simulink model "MotionControlRobuFastObsDynWithPredAdams2"  (Simulink 7.1)
settings: Solver=ode23  StartTime=0.0  StopTime=50  MaxStep=0.002  MinStep=0.0001  RelTol=0.2  AbsTol=0.1
StartFcn:
  | parameters
StopFcn:
  | replay
values from neighbouring files (symbols this model uses):
  ADAMS_cwd = '/home/roland/Bureau/Simulateur/SimulateurAdamsFaizRobuFASTB2'    [Controls_Plant_1.m]
  ADAMS_exec = ''    [Controls_Plant_1.m]
  ADAMS_host = 'krid.isir.upmc.fr'    [Controls_Plant_1.m]
  ADAMS_init = ''    [Controls_Plant_1.m]
  ADAMS_inputs = 'AngleBraquageAV!AngleBraquageArriere!AccelMoteur!Stab_function'    [Controls_Plant_1.m]
  ADAMS_outputs = 'PosX!PosY!PosXAvant!PosYAvant!MesureVitesse!AngleAVG!AngleAVD!AngleARG!AngleARD!VitesseRoueARD!VitesseRoueARG!VitesseLacet!roulis'    [Controls_Plant_1.m]
  ADAMS_prefix = 'Controls_Plant_1'    [Controls_Plant_1.m]
  ADAMS_static = 'yes'    [Controls_Plant_1.m]
  ADAMS_sysdir = '/home/roland/Adams/'    [Controls_Plant_1.m]
  C = ParDyn(9)    [MvtDyn.m]    (also in ParPneu.m = 1.3; Replay.m = line([X_trac(6) X_trac(8)],[Y_trac(6) Y_trac(8)],'LineWidth')
  Corr180 = Angle    [corr180.m]
undefined symbols (not defined in the file or in its folder): braquage2train2Arr, braquage3train2, CalculHorizonPred, courbure, DetDyn, ecarts, Empattement, MdresCarres, ObsCFCRMITtrain2, ObsDynTrain2, point_plus_proche, TrouvePos, Voie
libraries: simulink x8
(part 1 of 2)
settings Model: Creator=roland  LastModifiedBy=roland
settings SolverCC: InitialStep=0.001
settings DebuggingCC: SaveWithParameterizedLinksMsg=none  SignalResolutionControl=TryResolveAllWithWarning  MultiTaskDSMMsg=warning  MultiTaskCondExecSysMsg=none  StrictBusMsg=None
settings RTWCC: IncludeERTFirstTime=on
settings GRTTargetCC: TargetFcnLib=ansi_tfl_tmw.mat

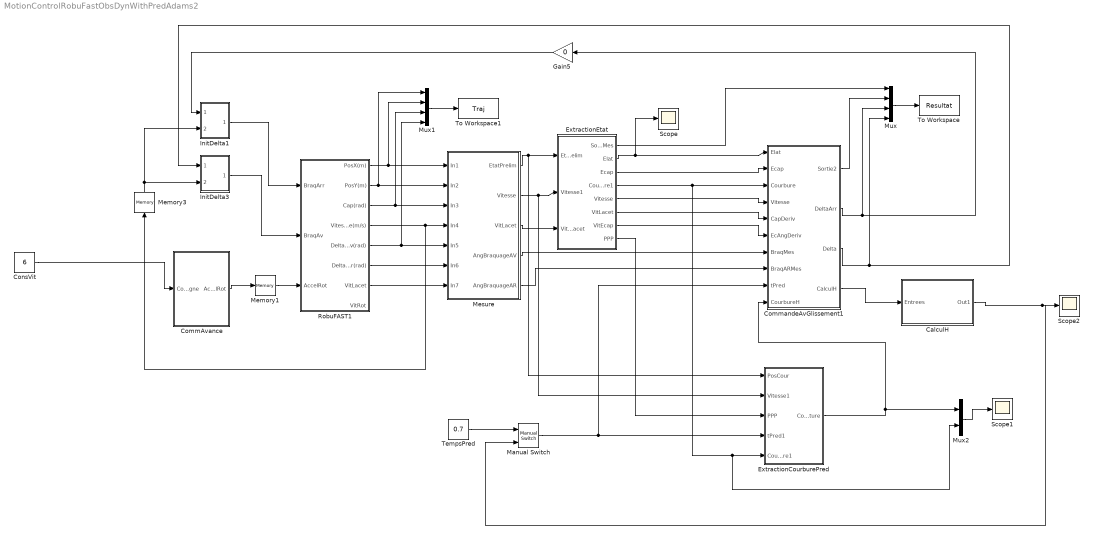
== system MotionControlRobuFastObsDynWithPredAdams2 ==
  CalculH : Subsystem
  CommAvance : Subsystem
  CommandeAvGlissement1 : Subsystem
  ConsVit : Constant  Value=6  OutDataType=sfix(16)  OutScaling=2^0
  ExtractionCourburePred : Subsystem
  ExtractionEtat : Subsystem
  Gain5 : Gain  Orientation=left  Gain=0  ParameterDataType=sfix(16)  ParameterScaling=2^0  OutDataType=sfix(16)  OutScaling=2^0
  InitDelta1 : Subsystem
  InitDelta3 : Subsystem
  Manual Switch : simulink/Signal Routing/Manual Switch  SystemSampleTime=-1  sw=1  action=0  varsize=off
  Memory1 : Memory  InheritSampleTime=on
  Memory3 : Memory  Orientation=up  InheritSampleTime=on
  Mesure : Subsystem
  Mux : Mux
  Mux1 : Mux
  Mux2 : Mux  Inputs=2
  RobuFAST1 : Subsystem
  Scope : Scope
      settings: TimeRange=25  YMin=-0.15  YMax=0.7  SaveName=Elat
  Scope1 : Scope
      settings: TimeRange=15  YMin=-1  YMax=1  SaveName=Elat1
  Scope2 : Scope
      settings: TimeRange=15  YMin=0.7245  YMax=0.7315  SaveName=Elat3
  TempsPred : Constant  Value=0.7  OutDataType=sfix(16)  OutScaling=2^0
  To Workspace : ToWorkspace  VariableName=Resultat  SampleTime=-1  SaveFormat=Array
  To Workspace1 : ToWorkspace  VariableName=Traj  SampleTime=-1  SaveFormat=Array
  wires:
  CommAvance/1(AccelRot) -> Memory1/1
  RobuFAST1/4(Vitesse(m/s)) -> Mesure/4(In4), Memory3/1
  RobuFAST1/1(PosX(m)) -> Mesure/1(In1), Mux1/2
  RobuFAST1/2(PosY(m)) -> Mesure/2(In2), Mux1/1
  RobuFAST1/3(Cap(rad)) -> Mesure/3(In3), Mux1/3
  Mesure/1(EtatPrelim) -> ExtractionEtat/1(EtatPrelim), ExtractionCourburePred/1(PosCour)
  Mesure/2(Vitesse) -> ExtractionEtat/2(Vitesse1), ExtractionCourburePred/2(Vitesse1)
  ExtractionEtat/2(Elat) -> Scope/1, CommandeAvGlissement1/1(Elat)
  ExtractionEtat/3(Ecap) -> CommandeAvGlissement1/2(Ecap)
  ExtractionEtat/4(Courbure1) -> CommandeAvGlissement1/3(Courbure), ExtractionCourburePred/5(Courbure1), Mux2/2
  ExtractionEtat/5(Vitesse) -> CommandeAvGlissement1/4(Vitesse)
  Mesure/4(AngBraquageAV) -> CommandeAvGlissement1/7(BraqMes)
  CommandeAvGlissement1/3(Delta) -> Mux/4, InitDelta3/1(Delta)
  CommandeAvGlissement1/2(DeltaArr) -> Gain5/1, Mux/3
  RobuFAST1/5(DeltaAv(rad)) -> Mesure/5(In5), Mux1/4
  RobuFAST1/6(DeltaAr(rad)) -> Mesure/6(In6)
  InitDelta1/1(Out1) -> RobuFAST1/1(BraqArr)
  InitDelta3/1(Out1) -> RobuFAST1/2(BraqAv)
  Memory3/1 -> InitDelta1/2(Vitesse), InitDelta3/2(Vitesse)
  Mesure/3(VitLacet) -> ExtractionEtat/3(VitesseLacet)
  ExtractionEtat/6(VitLacet) -> CommandeAvGlissement1/5(CapDeriv)
  RobuFAST1/7(VitLacet) -> Mesure/7(In7)
  ExtractionEtat/7(VitEcap) -> CommandeAvGlissement1/6(EcAngDeriv)
  ExtractionEtat/1(SortieMes) -> Mux/1
  CommandeAvGlissement1/1(Sortie2) -> Mux/2
  Mux/1 -> To Workspace/1
  Gain5/1 -> InitDelta1/1(Delta)
  Mux1/1 -> To Workspace1/1
  Mesure/5(AngBraquageAR) -> CommandeAvGlissement1/8(BraqARMes)
  Manual Switch/1 -> CommandeAvGlissement1/9(tPred), ExtractionCourburePred/4(tPred1)
  ExtractionCourburePred/1(CourbureFuture) -> CommandeAvGlissement1/10(CourbureH), Mux2/1
  ExtractionEtat/8(PPP) -> ExtractionCourburePred/3(PPP)
  Mux2/1 -> Scope1/1
  CalculH/1(Out1) -> Scope2/1, Manual Switch/2
  CommandeAvGlissement1/4(CalculH) -> CalculH/1(Entrees)
  ConsVit/1 -> CommAvance/1(Consigne)
  TempsPred/1 -> Manual Switch/1
  Memory1/1 -> RobuFAST1/3(AccelRot)

== system MotionControlRobuFastObsDynWithPredAdams2/CalculH ==
  Entrees : Inport
  CalculHorizonPred : MATLABFcn  MATLABFcn=CalculHorizonPred(u(1),u(2),u(3))  OutputDimensions=1  OutputSignalType=real  Output1D=off  SampleTime=0.05
  Discrete Filter8 : DiscreteFilter  Numerator=[0.025 0.025]  Denominator="[1.0000    -0.95]"  SampleTime=0.05
  Out1 : Outport
  wires:
  CalculHorizonPred/1 -> Out1/1
  Entrees/1 -> CalculHorizonPred/1

== system MotionControlRobuFastObsDynWithPredAdams2/CommAvance ==
  Consigne : Inport  OutDataType=sfix(16)  OutScaling=2^0
  Gain : Gain  Gain=1/0.25  ParameterDataType=sfix(16)  ParameterScaling=2^0  OutDataType=sfix(16)  OutScaling=2^0
  miseEnForme Condigne vitesse : Subsystem
  AccelRot : Outport  OutDataType=sfix(16)  OutScaling=2^0
  wires:
  miseEnForme Condigne vitesse/1(Out2) -> Gain/1
  Consigne/1 -> miseEnForme Condigne vitesse/1(In1)
  Gain/1 -> AccelRot/1

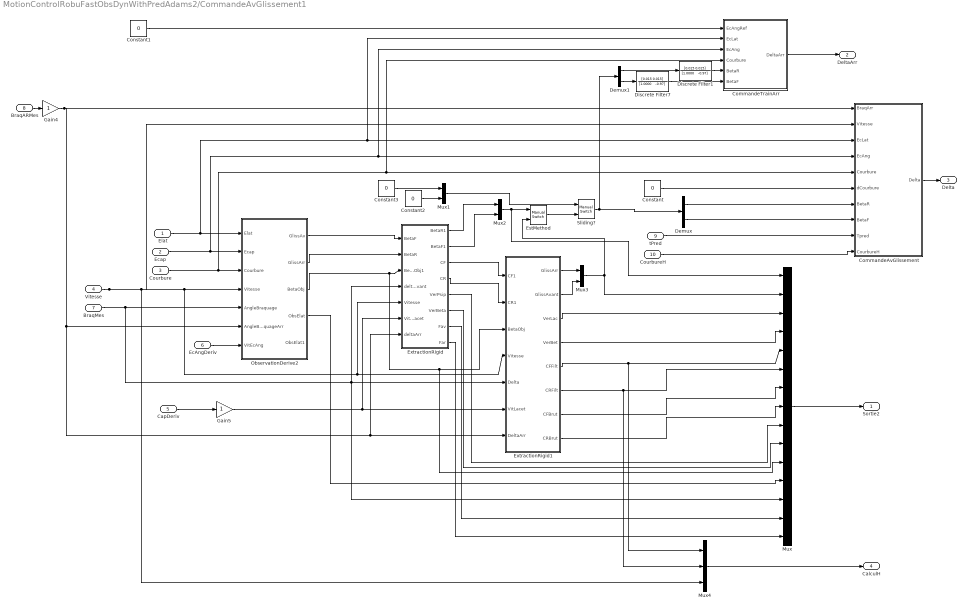
== system MotionControlRobuFastObsDynWithPredAdams2/CommandeAvGlissement1 ==
  Elat : Inport  OutDataType=sfix(16)  OutScaling=2^0
  Ecap : Inport  Port=2  OutDataType=sfix(16)  OutScaling=2^0
  Courbure : Inport  Port=3  OutDataType=sfix(16)  OutScaling=2^0
  Vitesse : Inport  Port=4  OutDataType=sfix(16)  OutScaling=2^0
  CapDeriv : Inport  Port=5  OutDataType=sfix(16)  OutScaling=2^0
  EcAngDeriv : Inport  Port=6  OutDataType=sfix(16)  OutScaling=2^0
  BraqMes : Inport  Port=7  OutDataType=sfix(16)  OutScaling=2^0
  BraqARMes : Inport  Port=8  OutDataType=sfix(16)  OutScaling=2^0
  tPred : Inport  Port=9  OutDataType=sfix(16)  OutScaling=2^0
  CourbureH : Inport  Port=10  OutDataType=sfix(16)  OutScaling=2^0
  CommandeAvGlissement : Subsystem
  CommandeTrainArr : Subsystem
  Constant{,1..3} (4 alike) : Constant  Value=0  OutDataType=sfix(16)  OutScaling=2^0
  Demux : Demux  Outputs=2
  Demux1 : Demux  Outputs=2
  Discrete Filter1 : DiscreteFilter  Numerator=[0.015 0.015]  Denominator="[1.0000    -0.97]"  SampleTime=0.05
  Discrete Filter7 : DiscreteFilter  Numerator=[0.015 0.015]  Denominator="[1.0000    -0.97]"  SampleTime=0.05
  EstMethod : simulink/Signal Routing/Manual Switch  SystemSampleTime=-1  sw=0  action=0  varsize=off
  ExtractionRigid : Subsystem
  ExtractionRigid1 : Subsystem
  Gain4 : Gain  ParameterDataType=sfix(16)  ParameterScaling=2^0  OutDataType=sfix(16)  OutScaling=2^0
  Gain5 : Gain  ParameterDataType=sfix(16)  ParameterScaling=2^0  OutDataType=sfix(16)  OutScaling=2^0
  Mux : Mux  Inputs=15
  Mux1 : Mux  Inputs=2
  Mux2 : Mux  Inputs=2
  Mux3 : Mux  Inputs=2
  Mux4 : Mux  Inputs=3
  ObservationDerive2 : Subsystem
  Sliding? : simulink/Signal Routing/Manual Switch  SystemSampleTime=-1  sw=0  action=0  varsize=off
  Sortie2 : Outport  OutDataType=sfix(16)  OutScaling=2^0
  DeltaArr : Outport  Port=2  OutDataType=sfix(16)  OutScaling=2^0
  Delta : Outport  Port=3  OutDataType=sfix(16)  OutScaling=2^0
  CalculH : Outport  Port=4  OutDataType=sfix(16)  OutScaling=2^0
  wires:
  BraqMes/1 -> ObservationDerive2/5(AngleBraquage), ExtractionRigid/4(deltaAvant), ExtractionRigid1/5(Delta), Mux/13
  Vitesse/1 -> CommandeAvGlissement/2(Vitesse), ObservationDerive2/4(Vitesse), ExtractionRigid/5(Vitesse), ExtractionRigid1/4(Vitesse), Mux4/3
  Constant/1 -> CommandeAvGlissement/6(dCourbure)
  Ecap/1 -> CommandeTrainArr/3(EcAng), CommandeAvGlissement/4(EcAng), ObservationDerive2/2(Ecap)
  Elat/1 -> CommandeTrainArr/2(EcLat), CommandeAvGlissement/3(EcLat), ObservationDerive2/1(Elat)
  Courbure/1 -> CommandeTrainArr/4(Courbure), CommandeAvGlissement/5(Courbure), ObservationDerive2/3(Courbure)
  BraqARMes/1 -> Gain4/1
  CommandeTrainArr/1(DeltaArr) -> DeltaArr/1
  Constant1/1 -> CommandeTrainArr/1(EcAngRef)
  Gain4/1 -> ObservationDerive2/6(AngleBraquageArr), ExtractionRigid1/7(DeltaArr), ExtractionRigid/7(deltaArr), CommandeAvGlissement/1(BraqArr)
  CapDeriv/1 -> Gain5/1
  Demux1/1 -> Discrete Filter1/1
  EcAngDeriv/1 -> ObservationDerive2/7(VitEcAng)
  ObservationDerive2/1(GlissAv) -> ExtractionRigid/1(BetaF)
  ObservationDerive2/2(GlissArr) -> ExtractionRigid/2(BetaR)
  Gain5/1 -> ExtractionRigid/6(VitesseLacet), ExtractionRigid1/6(VitLacet)
  ObservationDerive2/3(BetaObj) -> ExtractionRigid/3(BetaObj1), ExtractionRigid1/3(BetaObj), Mux/11
  Mux2/1 -> EstMethod/1, Mux/1
  Mux3/1 -> EstMethod/2, Mux/2
  Demux/2 -> CommandeAvGlissement/8(BetaF)
  Demux/1 -> CommandeAvGlissement/7(BetaR)
  Demux1/2 -> Discrete Filter7/1
  Discrete Filter7/1 -> CommandeTrainArr/6(BetaF)
  Discrete Filter1/1 -> CommandeTrainArr/5(BetaR)
  ExtractionRigid/2(BetaF1) -> Mux2/2
  ExtractionRigid/1(BetaR1) -> Mux2/1
  tPred/1 -> CommandeAvGlissement/9(Tpred)
  CourbureH/1 -> CommandeAvGlissement/10(CourbureH)
  ExtractionRigid1/1(GlissArr) -> Mux3/1
  ExtractionRigid1/2(GlissAvant) -> Mux3/2
  ExtractionRigid1/3(VerLac) -> Mux/3
  ExtractionRigid1/4(VerBet) -> Mux/4
  ExtractionRigid1/5(CFFilt) -> Mux/5, Mux4/1
  ExtractionRigid/4(CR) -> ExtractionRigid1/2(CR1)
  ExtractionRigid/5(VerPsip) -> Mux/9
  ObservationDerive2/4(ObsElat) -> Mux/12
  Mux/1 -> Sortie2/1
  ExtractionRigid/3(CF) -> ExtractionRigid1/1(CF1)
  ExtractionRigid1/6(CRFilt) -> Mux/6, Mux4/2
  ExtractionRigid1/7(CFBrut) -> Mux/7
  ExtractionRigid1/8(CRBrut) -> Mux/8
  ExtractionRigid/6(VerBeta) -> Mux/10
  Constant2/1 -> Mux1/2
  Constant3/1 -> Mux1/1
  Sliding?/1 -> Demux/1, Demux1/1
  EstMethod/1 -> Sliding?/2
  Mux1/1 -> Sliding?/1
  CommandeAvGlissement/1(Delta) -> Delta/1
  Mux4/1 -> CalculH/1
  ExtractionRigid/7(Fav) -> Mux/14
  ExtractionRigid/8(Far) -> Mux/15

== system MotionControlRobuFastObsDynWithPredAdams2/ExtractionCourburePred ==
  PosCour : Inport  OutDataType=sfix(16)  OutScaling=2^0
  Vitesse1 : Inport  Port=2  OutDataType=sfix(16)  OutScaling=2^0
  PPP : Inport  Port=3  OutDataType=sfix(16)  OutScaling=2^0
  tPred1 : Inport  Port=4  OutDataType=sfix(16)  OutScaling=2^0
  Courbure1 : Inport  Port=5  OutDataType=sfix(16)  OutScaling=2^0
  Courbure : MATLABFcn  MATLABFcn=courbure(u(1:3),u(4))  OutputDimensions=1  OutputSignalType=real  SampleTime=0.05
  MdreCarrees : MATLABFcn  MATLABFcn=MdresCarres(u(1:2),u(3))  OutputDimensions=3  OutputSignalType=real  SampleTime=0.05
  Mux1 : Mux  Inputs=2
  Mux3 : Mux  Inputs=2
  Mux4 : Mux  Inputs=5
  Point plus proche : Subsystem
  PosFuture : MATLABFcn  MATLABFcn=TrouvePos(u(1:3),u(4),u(5),u(6),u(7))  OutputDimensions=2  OutputSignalType=real  SampleTime=0.05
  CourbureFuture : Outport  OutDataType=sfix(16)  OutScaling=2^0
  wires:
  Vitesse1/1 -> Mux4/2
  Courbure/1 -> CourbureFuture/1
  Mux3/1 -> Courbure/1
  MdreCarrees/1 -> Mux3/1
  PosCour/1 -> Mux4/1
  PPP/1 -> Mux4/3
  tPred1/1 -> Mux4/4
  Mux4/1 -> PosFuture/1
  Courbure1/1 -> Mux4/5
  PosFuture/1 -> Point plus proche/1(In1), Mux1/1
  Point plus proche/1(Out1) -> Mux3/2, Mux1/2
  Mux1/1 -> MdreCarrees/1

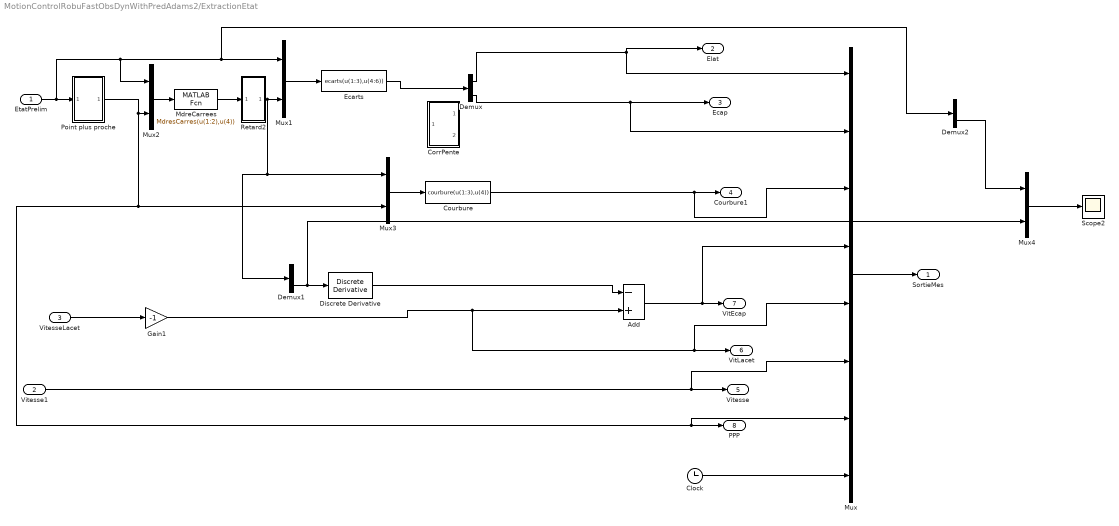
== system MotionControlRobuFastObsDynWithPredAdams2/ExtractionEtat ==
  EtatPrelim : Inport  OutDataType=sfix(16)  OutScaling=2^0
  Vitesse1 : Inport  Port=2  OutDataType=sfix(16)  OutScaling=2^0
  VitesseLacet : Inport  Port=3  OutDataType=sfix(16)  OutScaling=2^0
  Add : Sum  Inputs=-+  OutDataType=sfix(16)  OutScaling=2^-10
  Clock : Clock
      settings: Decimation=10
  CorrPente : Subsystem
  Courbure : MATLABFcn  MATLABFcn=courbure(u(1:3),u(4))  OutputDimensions=1  OutputSignalType=real  SampleTime=0.05
  Demux : Demux  Outputs=2
  Demux1 : Demux  Outputs=3
  Demux2 : Demux  Outputs=3
  Discrete Derivative : simulink/Discrete/Discrete Derivative  SystemSampleTime=-1  gainval=1.0  ICPrevScaledInput=0.0  OutMin=[]  OutMax=[]  OutDataType=sfix(16)  OutScaling=2^-10  DoSatur=off
  Ecarts : MATLABFcn  MATLABFcn=ecarts(u(1:3),u(4:6))  OutputDimensions=2  OutputSignalType=real  SampleTime=.05
  Gain1 : Gain  Gain=-1  ParameterDataType=sfix(16)  ParameterScaling=2^0  OutDataType=sfix(16)  OutScaling=2^0
  MdreCarrees : MATLABFcn  MATLABFcn=MdresCarres(u(1:2),u(4))  OutputDimensions=3  OutputSignalType=real  SampleTime=0.05
  Mux : Mux  Inputs=8
  Mux{1..4} (4 alike) : Mux  Inputs=2
  Point plus proche : Subsystem
  Retard2 : Subsystem
  Scope2 : Scope
      settings: TimeRange=15  YMin=-2.9  YMax=-1.5  SaveName=Elat4
  SortieMes : Outport  OutDataType=sfix(16)  OutScaling=2^0
  Elat : Outport  Port=2  OutDataType=sfix(16)  OutScaling=2^0
  Ecap : Outport  Port=3  OutDataType=sfix(16)  OutScaling=2^0
  Courbure1 : Outport  Port=4  OutDataType=sfix(16)  OutScaling=2^0
  Vitesse : Outport  Port=5  OutDataType=sfix(16)  OutScaling=2^0
  VitLacet : Outport  Port=6  OutDataType=sfix(16)  OutScaling=2^0
  VitEcap : Outport  Port=7  OutDataType=sfix(16)  OutScaling=2^0
  PPP : Outport  Port=8  OutDataType=sfix(16)  OutScaling=2^0
  wires:
  EtatPrelim/1 -> Mux2/1, Mux1/1, Demux2/1, Point plus proche/1(In1)
  Point plus proche/1(Out1) -> Mux2/2, Mux3/2, PPP/1, Mux/7
  Mux2/1 -> MdreCarrees/1
  Mux1/1 -> Ecarts/1
  Ecarts/1 -> Demux/1
  Mux3/1 -> Courbure/1
  Courbure/1 -> Courbure1/1, Mux/3
  Vitesse1/1 -> Vitesse/1, Mux/6
  MdreCarrees/1 -> Retard2/1(In1)
  Demux1/3 -> Discrete Derivative/1, Mux4/2
  VitesseLacet/1 -> Gain1/1
  Gain1/1 -> Add/2, VitLacet/1, Mux/5
  Discrete Derivative/1 -> Add/1
  Add/1 -> VitEcap/1, Mux/4
  Clock/1 -> Mux/8
  Mux/1 -> SortieMes/1
  Demux/1 -> Elat/1, Mux/1
  Demux2/3 -> Mux4/1
  Mux4/1 -> Scope2/1
  Demux/2 -> Ecap/1, Mux/2
  Retard2/1(Out1) -> Mux1/2, Mux3/1, Demux1/1

== system MotionControlRobuFastObsDynWithPredAdams2/InitDelta1 ==
  Delta : Inport  OutDataType=sfix(16)  OutScaling=2^0
  Vitesse : Inport  Port=2  OutDataType=sfix(16)  OutScaling=2^0
  Clock : Clock
      settings: Decimation=10
  Constant1 : Constant  Value=0  OutDataType=sfix(16)  OutScaling=2^0
  Constant2 : Constant  Value=0  OutDataType=sfix(16)  OutScaling=2^0
  Discrete Filter1 : DiscreteFilter  Numerator=[0.2167 0.1485]  Denominator=[1 -0.9610 0.3263]  SampleTime=.02
  Discrete Filter2 : DiscreteFilter  Numerator=[0.1 0.1]  Denominator=[1 -0.8]  SampleTime=.05
  Memory1 : Memory  InheritSampleTime=on
  Memory2 : Memory  InheritSampleTime=on
  Switch1 : Switch  Threshold=1  SaturateOnIntegerOverflow=on
  Switch2 : Switch  Threshold=2.5  SaturateOnIntegerOverflow=on
  Transfer Fcn : TransferFcn  Numerator=[80]  Denominator=[1 13 80]
  Zero-Order Hold : ZeroOrderHold  SampleTime=0.05
  Out1 : Outport  OutDataType=sfix(16)  OutScaling=2^0
  wires:
  Zero-Order Hold/1 -> Memory1/1
  Memory2/1 -> Transfer Fcn/1
  Memory1/1 -> Memory2/1
  Switch2/1 -> Zero-Order Hold/1
  Switch1/1 -> Switch2/1
  Constant2/1 -> Switch2/3
  Clock/1 -> Switch2/2
  Vitesse/1 -> Switch1/2
  Transfer Fcn/1 -> Out1/1
  Delta/1 -> Switch1/1
  Constant1/1 -> Switch1/3

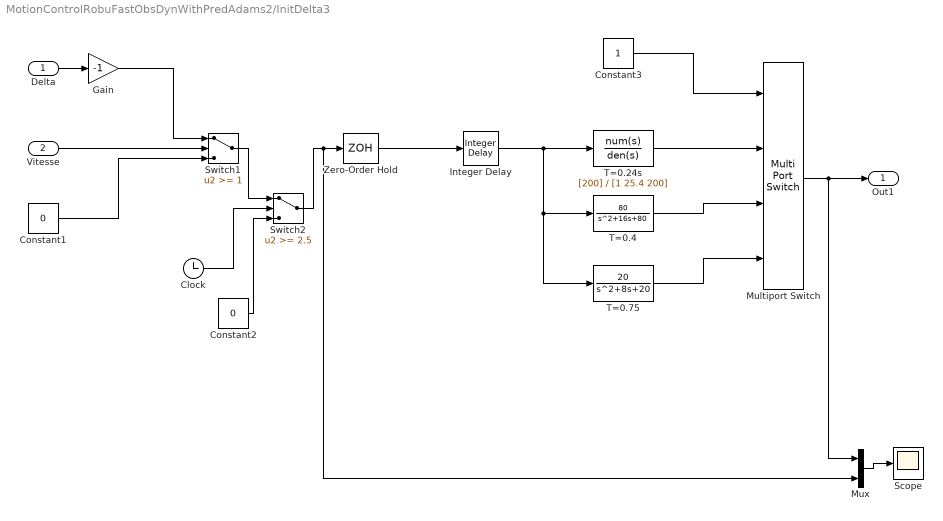
== system MotionControlRobuFastObsDynWithPredAdams2/InitDelta3 ==
  Delta : Inport  OutDataType=sfix(16)  OutScaling=2^0
  Vitesse : Inport  Port=2  OutDataType=sfix(16)  OutScaling=2^0
  Clock : Clock
      settings: Decimation=10
  Constant1 : Constant  Value=0  OutDataType=sfix(16)  OutScaling=2^0
  Constant2 : Constant  Value=0  OutDataType=sfix(16)  OutScaling=2^0
  Constant3 : Constant  OutDataType=sfix(16)  OutScaling=2^0
  Gain : Gain  Gain=-1  ParameterDataType=sfix(16)  ParameterScaling=2^0  OutDataType=sfix(16)  OutScaling=2^0
  Integer Delay : simulink/Discrete/Integer Delay  vinit=0.0  samptime=-1  NumDelays=2
  Multiport Switch : MultiPortSwitch
  Mux : Mux  Inputs=2
  Scope : Scope
      settings: YMin=-0.05  YMax=0.25  SaveName=ScopeData7
  Switch1 : Switch  Threshold=1  SaturateOnIntegerOverflow=on
  Switch2 : Switch  Threshold=2.5  SaturateOnIntegerOverflow=on
  T=0.24s : TransferFcn  Numerator=[200]  Denominator=[1 25.4 200]
  T=0.4 : TransferFcn  Numerator=[80]  Denominator=[1 16 80]
  T=0.75 : TransferFcn  Numerator=[20]  Denominator=[1 8 20]
  Zero-Order Hold : ZeroOrderHold  SampleTime=0.05
  Out1 : Outport  OutDataType=sfix(16)  OutScaling=2^0
  wires:
  Constant1/1 -> Switch1/3
  Delta/1 -> Gain/1
  Vitesse/1 -> Switch1/2
  Clock/1 -> Switch2/2
  Constant2/1 -> Switch2/3
  Switch1/1 -> Switch2/1
  Switch2/1 -> Zero-Order Hold/1, Mux/2
  T=0.24s/1 -> Multiport Switch/2
  T=0.4/1 -> Multiport Switch/3
  T=0.75/1 -> Multiport Switch/4
  Multiport Switch/1 -> Out1/1, Mux/1
  Constant3/1 -> Multiport Switch/1
  Zero-Order Hold/1 -> Integer Delay/1
  Mux/1 -> Scope/1
  Integer Delay/1 -> T=0.24s/1, T=0.4/1, T=0.75/1
  Gain/1 -> Switch1/1

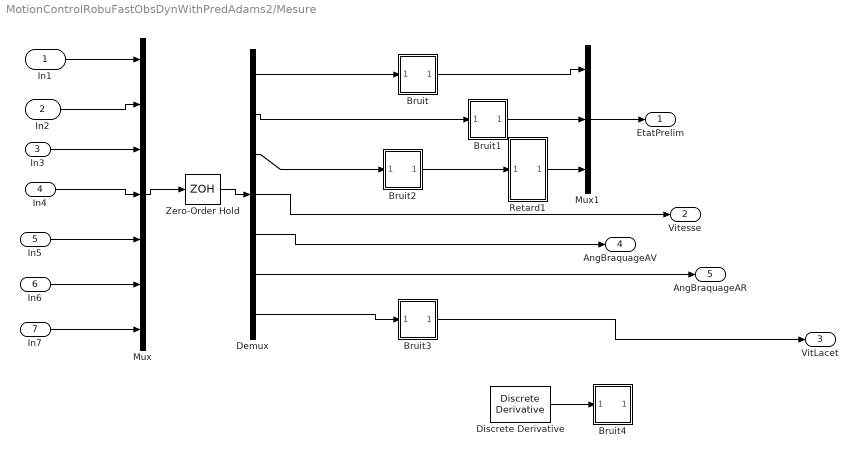
== system MotionControlRobuFastObsDynWithPredAdams2/Mesure ==
  In1 : Inport  OutDataType=sfix(16)  OutScaling=2^0
  In2 : Inport  Port=2  OutDataType=sfix(16)  OutScaling=2^0
  In3 : Inport  Port=3  OutDataType=sfix(16)  OutScaling=2^0
  In4 : Inport  Port=4  OutDataType=sfix(16)  OutScaling=2^0
  In5 : Inport  Port=5  OutDataType=sfix(16)  OutScaling=2^0
  In6 : Inport  Port=6  OutDataType=sfix(16)  OutScaling=2^0
  In7 : Inport  Port=7  OutDataType=sfix(16)  OutScaling=2^0
  Bruit : Subsystem
  Bruit1 : Subsystem
  Bruit2 : Subsystem
  Bruit3 : Subsystem
  Bruit4 : Subsystem
  Demux : Demux  Outputs=7
  Discrete Derivative : simulink/Discrete/Discrete Derivative  SystemSampleTime=-1  gainval=-1.0  ICPrevScaledInput=0.0  OutMin=[]  OutMax=[]  OutDataType=sfix(16)  OutScaling=2^-10  DoSatur=off
  Mux : Mux  Inputs=7
  Mux1 : Mux  Inputs=3
  Retard1 : Subsystem
  Zero-Order Hold : ZeroOrderHold  SampleTime=0.05
  EtatPrelim : Outport  OutDataType=sfix(16)  OutScaling=2^0
  Vitesse : Outport  Port=2  OutDataType=sfix(16)  OutScaling=2^0
  VitLacet : Outport  Port=3  OutDataType=sfix(16)  OutScaling=2^0
  AngBraquageAV : Outport  Port=4  OutDataType=sfix(16)  OutScaling=2^0
  AngBraquageAR : Outport  Port=5  OutDataType=sfix(16)  OutScaling=2^0
  wires:
  Mux1/1 -> EtatPrelim/1
  Zero-Order Hold/1 -> Demux/1
  Mux/1 -> Zero-Order Hold/1
  In1/1 -> Mux/1
  In2/1 -> Mux/2
  In3/1 -> Mux/3
  In4/1 -> Mux/4
  In5/1 -> Mux/5
  In6/1 -> Mux/6
  Demux/1 -> Bruit/1(In1)
  Demux/2 -> Bruit1/1(In1)
  Demux/3 -> Bruit2/1(In1)
  Demux/4 -> Vitesse/1
  Demux/5 -> AngBraquageAV/1
  Demux/6 -> AngBraquageAR/1
  Demux/7 -> Bruit3/1(In1)
  In7/1 -> Mux/7
  Bruit/1(Out1) -> Mux1/1
  Bruit1/1(Out1) -> Mux1/2
  Bruit2/1(Out1) -> Retard1/1(In1)
  Discrete Derivative/1 -> Bruit4/1(In1)
  Bruit3/1(Out1) -> VitLacet/1
  Retard1/1(Out1) -> Mux1/3

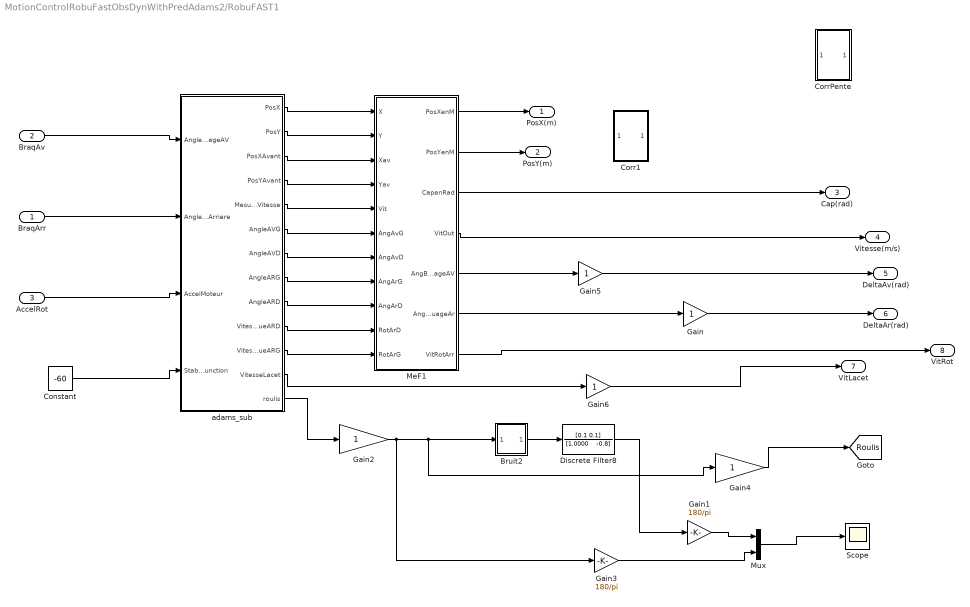
== system MotionControlRobuFastObsDynWithPredAdams2/RobuFAST1 ==
  BraqArr : Inport  OutDataType=sfix(16)  OutScaling=2^0
  BraqAv : Inport  Port=2  OutDataType=sfix(16)  OutScaling=2^0
  AccelRot : Inport  Port=3  OutDataType=sfix(16)  OutScaling=2^0
  Bruit2 : Subsystem
  Constant : Constant  Value=-60  OutDataType=sfix(16)  OutScaling=2^0
  Corr1 : Subsystem
  CorrPente : Subsystem
  Discrete Filter8 : DiscreteFilter  Numerator=[0.1 0.1]  Denominator="[1.0000    -0.8]"  SampleTime=0.05
  Gain{,2,4..6} (5 alike) : Gain  ParameterDataType=sfix(16)  ParameterScaling=2^0  OutDataType=sfix(16)  OutScaling=2^0
  Gain1 : Gain  Gain=180/pi  ParameterDataType=sfix(16)  ParameterScaling=2^0  OutDataType=sfix(16)  OutScaling=2^0
  Gain3 : Gain  Gain=180/pi  ParameterDataType=sfix(16)  ParameterScaling=2^0  OutDataType=sfix(16)  OutScaling=2^0
  MeF1 : Subsystem
  Mux : Mux  Inputs=2
  Scope : Scope
      settings: TimeRange=16  YMin=-10  YMax=2
  adams_sub : Subsystem
  PosX(m) : Outport  OutDataType=sfix(16)  OutScaling=2^0
  PosY(m) : Outport  Port=2  OutDataType=sfix(16)  OutScaling=2^0
  Cap(rad) : Outport  Port=3  OutDataType=sfix(16)  OutScaling=2^0
  Vitesse(m/s) : Outport  Port=4  OutDataType=sfix(16)  OutScaling=2^0
  DeltaAv(rad) : Outport  Port=5  OutDataType=sfix(16)  OutScaling=2^0
  DeltaAr(rad) : Outport  Port=6  OutDataType=sfix(16)  OutScaling=2^0
  VitLacet : Outport  Port=7  OutDataType=sfix(16)  OutScaling=2^0
  VitRot : Outport  Port=8  OutDataType=sfix(16)  OutScaling=2^0
  tag scope: Roulis=global
  wires:
  MeF1/1(PosXenM) -> PosX(m)/1
  BraqAv/1 -> adams_sub/1("AngleBraquageAV     ")
  MeF1/2(PosYenM) -> PosY(m)/1
  MeF1/4(VitOut) -> Vitesse(m/s)/1
  BraqArr/1 -> adams_sub/2(AngleBraquageArriere)
  MeF1/5(AngBraquageAV) -> Gain5/1
  MeF1/6(AngBraquageAr) -> Gain/1
  AccelRot/1 -> adams_sub/3("AccelMoteur         ")
  MeF1/7(VitRotArr) -> VitRot/1
  adams_sub/1("PosX          ") -> MeF1/1(X)
  adams_sub/2("PosY          ") -> MeF1/2(Y)
  adams_sub/3("PosXAvant     ") -> MeF1/3(Xav)
  adams_sub/4("PosYAvant     ") -> MeF1/4(Yav)
  adams_sub/5("MesureVitesse ") -> MeF1/5(Vit)
  adams_sub/6("AngleAVG      ") -> MeF1/6(AngAvG)
  adams_sub/7("AngleAVD      ") -> MeF1/7(AngAvD)
  adams_sub/8("AngleARG      ") -> MeF1/8(AngArG)
  adams_sub/9("AngleARD      ") -> MeF1/9(AngArD)
  adams_sub/10(VitesseRoueARD) -> MeF1/10(RotArD)
  adams_sub/11(VitesseRoueARG) -> MeF1/11(RotArG)
  MeF1/3(CapenRad) -> Cap(rad)/1
  adams_sub/13("roulis        ") -> Gain2/1
  Gain2/1 -> Gain3/1, Bruit2/1(In1), Gain4/1
  Bruit2/1(Out1) -> Discrete Filter8/1
  Discrete Filter8/1 -> Gain1/1
  Gain1/1 -> Mux/1
  Mux/1 -> Scope/1
  Gain3/1 -> Mux/2
  adams_sub/12("VitesseLacet  ") -> Gain6/1
  Gain4/1 -> [Roulis]
  Constant/1 -> adams_sub/4("Stab_function       ")
  Gain/1 -> DeltaAr(rad)/1
  Gain5/1 -> DeltaAv(rad)/1
  Gain6/1 -> VitLacet/1

== system MotionControlRobuFastObsDynWithPredAdams2/CommAvance/miseEnForme Condigne vitesse ==
  In1 : Inport  OutDataType=sfix(16)  OutScaling=2^0
  Braquage2 : Constant  Value=0  OutDataType=sfix(16)  OutScaling=2^0
  Clock : Clock
      settings: Decimation=10
  Switch : Switch  Threshold=1.5
  T=0.75 : TransferFcn  Numerator=[20]  Denominator=[1 8 20]
  Out2 : Outport  OutDataType=sfix(16)  OutScaling=2^0
  wires:
  T=0.75/1 -> Out2/1
  Clock/1 -> Switch/2
  Braquage2/1 -> Switch/3
  Switch/1 -> T=0.75/1
  In1/1 -> Switch/1

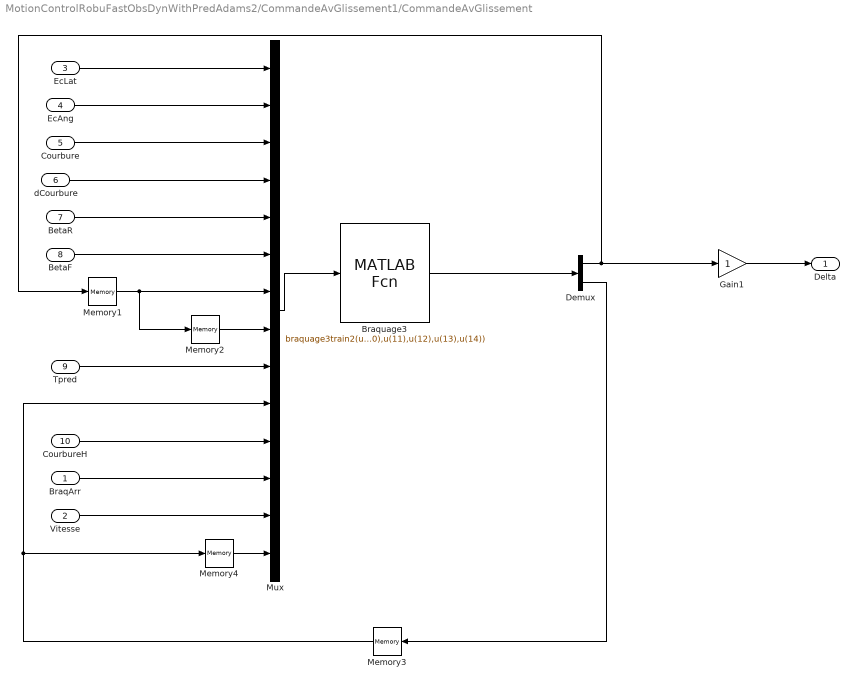
== system MotionControlRobuFastObsDynWithPredAdams2/CommandeAvGlissement1/CommandeAvGlissement ==
  BraqArr : Inport  OutDataType=sfix(16)  OutScaling=2^0
  Vitesse : Inport  Port=2  OutDataType=sfix(16)  OutScaling=2^0
  EcLat : Inport  Port=3  OutDataType=sfix(16)  OutScaling=2^0
  EcAng : Inport  Port=4  OutDataType=sfix(16)  OutScaling=2^0
  Courbure : Inport  Port=5  OutDataType=sfix(16)  OutScaling=2^0
  dCourbure : Inport  Port=6  OutDataType=sfix(16)  OutScaling=2^0
  BetaR : Inport  Port=7  OutDataType=sfix(16)  OutScaling=2^0
  BetaF : Inport  Port=8  OutDataType=sfix(16)  OutScaling=2^0
  Tpred : Inport  Port=9  OutDataType=sfix(16)  OutScaling=2^0
  CourbureH : Inport  Port=10  OutDataType=sfix(16)  OutScaling=2^0
  Braquage3 : MATLABFcn  MATLABFcn=braquage3train2(u(1),u(2),u(3),u(4),u(5),u(6),u(7),u(8),u(9),u(10),u(11),u(12),u(13),u(14))  OutputDimensions=2  OutputSignalType=real  SampleTime=0.05
  Demux : Demux  Outputs=2
  Gain1 : Gain  ParameterDataType=sfix(16)  ParameterScaling=2^0  OutDataType=sfix(16)  OutScaling=2^0
  Memory1 : Memory  InheritSampleTime=on
  Memory2 : Memory  InheritSampleTime=on
  Memory3 : Memory  Orientation=left  InheritSampleTime=on
  Memory4 : Memory  InheritSampleTime=on
  Mux : Mux  Inputs=14
  Delta : Outport  OutDataType=sfix(16)  OutScaling=2^0
  wires:
  BetaR/1 -> Mux/5
  BetaF/1 -> Mux/6
  dCourbure/1 -> Mux/4
  Gain1/1 -> Delta/1
  Courbure/1 -> Mux/3
  EcAng/1 -> Mux/2
  EcLat/1 -> Mux/1
  Mux/1 -> Braquage3/1
  Tpred/1 -> Mux/9
  CourbureH/1 -> Mux/11
  Memory1/1 -> Mux/7, Memory2/1
  Memory2/1 -> Mux/8
  Braquage3/1 -> Demux/1
  Demux/1 -> Gain1/1, Memory1/1
  Demux/2 -> Memory3/1
  BraqArr/1 -> Mux/12
  Memory3/1 -> Mux/10, Memory4/1
  Vitesse/1 -> Mux/13
  Memory4/1 -> Mux/14

== system MotionControlRobuFastObsDynWithPredAdams2/CommandeAvGlissement1/CommandeTrainArr ==
  EcAngRef : Inport  OutDataType=sfix(16)  OutScaling=2^0
  EcLat : Inport  Port=2  OutDataType=sfix(16)  OutScaling=2^0
  EcAng : Inport  Orientation=up  Port=3  OutDataType=sfix(16)  OutScaling=2^0
  Courbure : Inport  Port=4  OutDataType=sfix(16)  OutScaling=2^0
  BetaR : Inport  Port=5  OutDataType=sfix(16)  OutScaling=2^0
  BetaF : Inport  Port=6  OutDataType=sfix(16)  OutScaling=2^0
  Braquage2train2Arr : MATLABFcn  MATLABFcn=braquage2train2Arr(u(1),u(2),u(3),u(4),u(5),u(6))  OutputDimensions=1  OutputSignalType=real  SampleTime=0.05
  Gain1 : Gain  Gain=0  ParameterDataType=sfix(16)  ParameterScaling=2^0  OutDataType=sfix(16)  OutScaling=2^0
  Gain2 : Gain  Gain=pi/180  ParameterDataType=sfix(16)  ParameterScaling=2^0  OutDataType=sfix(16)  OutScaling=2^0
  Mux : Mux  Inputs=6
  DeltaArr : Outport  OutDataType=sfix(16)  OutScaling=2^0
  wires:
  EcAngRef/1 -> Gain2/1
  Mux/1 -> Braquage2train2Arr/1
  Braquage2train2Arr/1 -> Gain1/1
  EcLat/1 -> Mux/1
  EcAng/1 -> Mux/2
  Courbure/1 -> Mux/3
  Gain1/1 -> DeltaArr/1
  Gain2/1 -> Mux/6
  BetaR/1 -> Mux/4
  BetaF/1 -> Mux/5

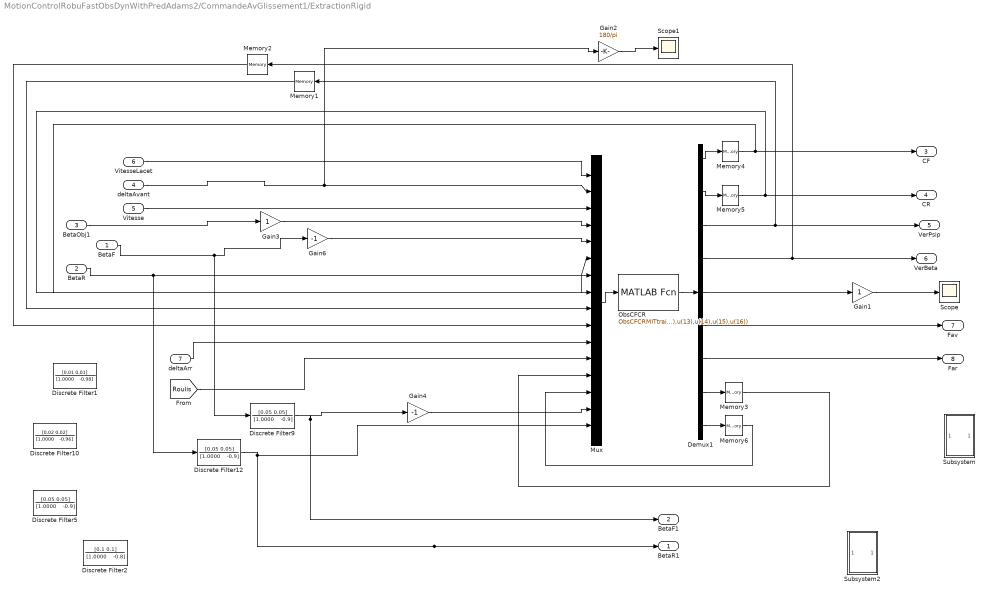
== system MotionControlRobuFastObsDynWithPredAdams2/CommandeAvGlissement1/ExtractionRigid ==
  BetaF : Inport  OutDataType=sfix(16)  OutScaling=2^0
  BetaR : Inport  Port=2  OutDataType=sfix(16)  OutScaling=2^0
  BetaObj1 : Inport  Port=3  OutDataType=sfix(16)  OutScaling=2^0
  deltaAvant : Inport  Port=4  OutDataType=sfix(16)  OutScaling=2^0
  Vitesse : Inport  Port=5  OutDataType=sfix(16)  OutScaling=2^0
  VitesseLacet : Inport  Port=6  OutDataType=sfix(16)  OutScaling=2^0
  deltaArr : Inport  Port=7  OutDataType=sfix(16)  OutScaling=2^0
  Demux1 : Demux  Outputs=9
  Discrete Filter1 : DiscreteFilter  Numerator=[0.01 0.01]  Denominator="[1.0000    -0.98]"  SampleTime=0.05
  Discrete Filter10 : DiscreteFilter  Numerator=[0.02 0.02]  Denominator="[1.0000    -0.96]"  SampleTime=0.05
  Discrete Filter12 : DiscreteFilter  Numerator=[0.05 0.05]  Denominator="[1.0000    -0.9]"  SampleTime=0.05
  Discrete Filter2 : DiscreteFilter  Numerator=[0.1 0.1]  Denominator="[1.0000    -0.8]"  SampleTime=0.05
  Discrete Filter5 : DiscreteFilter  Numerator=[0.05 0.05]  Denominator="[1.0000    -0.9]"  SampleTime=0.05
  Discrete Filter9 : DiscreteFilter  Numerator=[0.05 0.05]  Denominator="[1.0000    -0.9]"  SampleTime=0.05
  Gain1 : Gain  ParameterDataType=sfix(16)  ParameterScaling=2^0  OutDataType=sfix(16)  OutScaling=2^0
  Gain2 : Gain  Gain=180/pi  ParameterDataType=sfix(16)  ParameterScaling=2^0  OutDataType=sfix(16)  OutScaling=2^0
  Gain3 : Gain  ParameterDataType=sfix(16)  ParameterScaling=2^0  OutDataType=sfix(16)  OutScaling=2^0
  Gain4 : Gain  Gain=-1  ParameterDataType=sfix(16)  ParameterScaling=2^0  OutDataType=sfix(16)  OutScaling=2^0
  Gain6 : Gain  Gain=-1  ParameterDataType=sfix(16)  ParameterScaling=2^0  OutDataType=sfix(16)  OutScaling=2^0
  Memory1 : Memory  Orientation=left  InheritSampleTime=on
  Memory2 : Memory  Orientation=left  InheritSampleTime=on
  Memory3 : Memory  InheritSampleTime=on
  Memory4 : Memory  X0=5000  InheritSampleTime=on
  Memory5 : Memory  X0=5000  InheritSampleTime=on
  Memory6 : Memory  InheritSampleTime=on
  Mux : Mux  Inputs=16
  ObsCFCR : MATLABFcn  MATLABFcn=ObsCFCRMITtrain2(u(1),u(2),u(3),u(4),u(5),u(6),u(7),u(8),u(9),u(10),u(11),u(12),u(13),u(14),u(15),u(16))  OutputDimensions=9  OutputSignalType=real  SampleTime=0.05
  Scope : Scope
      settings: TimeRange=10  YMin=200  YMax=200  SaveName=ScopeData6
  Scope1 : Scope
      settings: TimeRange=10  YMin=0  YMax=35000  SaveName=ScopeData5
  Subsystem : Subsystem
  Subsystem2 : Subsystem
  BetaR1 : Outport  OutDataType=sfix(16)  OutScaling=2^0
  BetaF1 : Outport  Port=2  OutDataType=sfix(16)  OutScaling=2^0
  CF : Outport  Port=3  OutDataType=sfix(16)  OutScaling=2^0
  CR : Outport  Port=4  OutDataType=sfix(16)  OutScaling=2^0
  VerPsip : Outport  Port=5  OutDataType=sfix(16)  OutScaling=2^0
  VerBeta : Outport  Port=6  OutDataType=sfix(16)  OutScaling=2^0
  Fav : Outport  Port=7  OutDataType=sfix(16)  OutScaling=2^0
  Far : Outport  Port=8  OutDataType=sfix(16)  OutScaling=2^0
  wires:
  ObsCFCR/1 -> Demux1/1
  Mux/1 -> ObsCFCR/1
  Demux1/1 -> Memory4/1
  Demux1/2 -> Memory5/1
  VitesseLacet/1 -> Mux/1
  deltaAvant/1 -> Mux/2, Gain2/1
  Vitesse/1 -> Mux/3
  BetaObj1/1 -> Gain3/1
  Demux1/3 -> Memory1/1, VerPsip/1
  Demux1/4 -> Memory2/1, VerBeta/1
  BetaF/1 -> Discrete Filter9/1, Gain6/1
  BetaR/1 -> Discrete Filter12/1, Mux/6
  Memory1/1 -> Mux/9
  Memory2/1 -> Mux/10
  Memory4/1 -> CF/1, Mux/7
  Memory5/1 -> Mux/8, CR/1
  Demux1/5 -> Gain1/1
  Gain6/1 -> Mux/5
  deltaArr/1 -> Mux/11
  [Roulis] -> Mux/12
  Gain1/1 -> Scope/1
  Demux1/6 -> Fav/1
  Demux1/7 -> Far/1
  Demux1/8 -> Memory3/1
  Memory3/1 -> Mux/13
  Demux1/9 -> Memory6/1
  Memory6/1 -> Mux/14
  Discrete Filter9/1 -> BetaF1/1, Gain4/1
  Discrete Filter12/1 -> BetaR1/1, Mux/16
  Gain2/1 -> Scope1/1
  Gain3/1 -> Mux/4
  Gain4/1 -> Mux/15

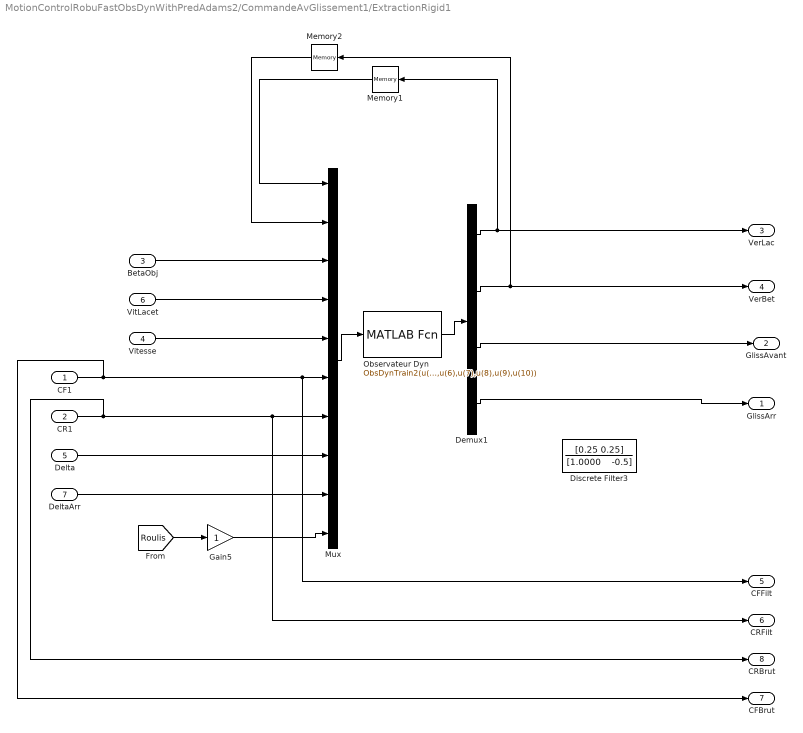
== system MotionControlRobuFastObsDynWithPredAdams2/CommandeAvGlissement1/ExtractionRigid1 ==
  CF1 : Inport  OutDataType=sfix(16)  OutScaling=2^0
  CR1 : Inport  Port=2  OutDataType=sfix(16)  OutScaling=2^0
  BetaObj : Inport  Port=3  OutDataType=sfix(16)  OutScaling=2^0
  Vitesse : Inport  Port=4  OutDataType=sfix(16)  OutScaling=2^0
  Delta : Inport  Port=5  OutDataType=sfix(16)  OutScaling=2^0
  VitLacet : Inport  Port=6  OutDataType=sfix(16)  OutScaling=2^0
  DeltaArr : Inport  Port=7  OutDataType=sfix(16)  OutScaling=2^0
  Demux1 : Demux
  Discrete Filter3 : DiscreteFilter  Numerator=[0.25 0.25]  Denominator="[1.0000    -0.5]"  SampleTime=0.05
  Gain5 : Gain  ParameterDataType=sfix(16)  ParameterScaling=2^0  OutDataType=sfix(16)  OutScaling=2^0
  Memory1 : Memory  Orientation=left  InheritSampleTime=on
  Memory2 : Memory  Orientation=left  InheritSampleTime=on
  Mux : Mux  Inputs=10
  Observateur Dyn : MATLABFcn  MATLABFcn=ObsDynTrain2(u(1),u(2),u(3),u(4),u(5),u(6),u(7),u(8),u(9),u(10))  OutputDimensions=4  OutputSignalType=real  SampleTime=0.05
  GlissArr : Outport  OutDataType=sfix(16)  OutScaling=2^0
  GlissAvant : Outport  Port=2  OutDataType=sfix(16)  OutScaling=2^0
  VerLac : Outport  Port=3  OutDataType=sfix(16)  OutScaling=2^0
  VerBet : Outport  Port=4  OutDataType=sfix(16)  OutScaling=2^0
  CFFilt : Outport  Port=5  OutDataType=sfix(16)  OutScaling=2^0
  CRFilt : Outport  Port=6  OutDataType=sfix(16)  OutScaling=2^0
  CFBrut : Outport  Port=7  OutDataType=sfix(16)  OutScaling=2^0
  CRBrut : Outport  Port=8  OutDataType=sfix(16)  OutScaling=2^0
  wires:
  Demux1/4 -> GlissArr/1
  Demux1/3 -> GlissAvant/1
  Demux1/2 -> VerBet/1, Memory2/1
  Demux1/1 -> VerLac/1, Memory1/1
  Mux/1 -> Observateur Dyn/1
  Observateur Dyn/1 -> Demux1/1
  Memory1/1 -> Mux/1
  Memory2/1 -> Mux/2
  BetaObj/1 -> Mux/3
  VitLacet/1 -> Mux/4
  Vitesse/1 -> Mux/5
  CF1/1 -> CFBrut/1, Mux/6, CFFilt/1
  CR1/1 -> CRBrut/1, Mux/7, CRFilt/1
  Delta/1 -> Mux/8
  DeltaArr/1 -> Mux/9
  [Roulis] -> Gain5/1
  Gain5/1 -> Mux/10

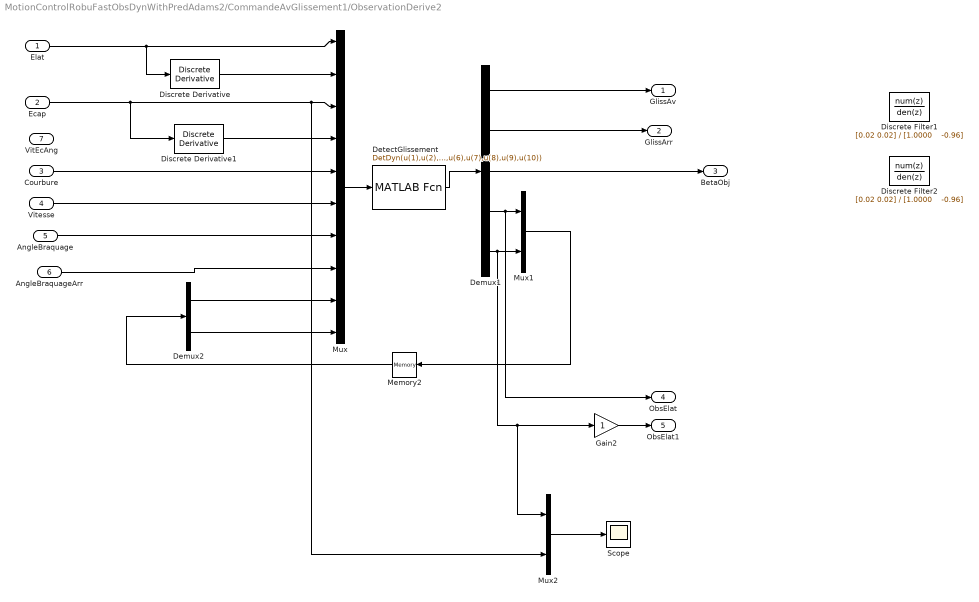
== system MotionControlRobuFastObsDynWithPredAdams2/CommandeAvGlissement1/ObservationDerive2 ==
  Elat : Inport  OutDataType=sfix(16)  OutScaling=2^0
  Ecap : Inport  Port=2  OutDataType=sfix(16)  OutScaling=2^0
  Courbure : Inport  Port=3  OutDataType=sfix(16)  OutScaling=2^0
  Vitesse : Inport  Port=4  OutDataType=sfix(16)  OutScaling=2^0
  AngleBraquage : Inport  Port=5  OutDataType=sfix(16)  OutScaling=2^0
  AngleBraquageArr : Inport  Port=6  OutDataType=sfix(16)  OutScaling=2^0
  VitEcAng : Inport  Port=7  OutDataType=sfix(16)  OutScaling=2^0
  Demux1 : Demux  Outputs=5
  Demux2 : Demux  Outputs=2
  DetectGlissement : MATLABFcn  MATLABFcn=DetDyn(u(1),u(2),u(3),u(4),u(5),u(6),u(7),u(8),u(9),u(10))  OutputDimensions=5  OutputSignalType=real  SampleTime=0.05
  Discrete Derivative : simulink/Discrete/Discrete Derivative  SystemSampleTime=-1  gainval=1.0  ICPrevScaledInput=0.0  OutMin=[]  OutMax=[]  OutDataType=sfix(16)  OutScaling=2^-10  DoSatur=off
  Discrete Derivative1 : simulink/Discrete/Discrete Derivative  SystemSampleTime=-1  gainval=1.0  ICPrevScaledInput=0.0  OutMin=[]  OutMax=[]  OutDataType=sfix(16)  OutScaling=2^-10  DoSatur=off
  Discrete Filter1 : DiscreteFilter  Numerator=[0.02 0.02]  Denominator="[1.0000    -0.96]"  SampleTime=0.05
  Discrete Filter2 : DiscreteFilter  Numerator=[0.02 0.02]  Denominator="[1.0000    -0.96]"  SampleTime=0.05
  Gain2 : Gain  ParameterDataType=sfix(16)  ParameterScaling=2^0  OutDataType=sfix(16)  OutScaling=2^0
  Memory2 : Memory  Orientation=left  InheritSampleTime=on
  Mux : Mux  Inputs=10
  Mux1 : Mux  Inputs=2
  Mux2 : Mux  Inputs=2
  Scope : Scope
      settings: YMin=-0.175  YMax=0.15
  GlissAv : Outport  OutDataType=sfix(16)  OutScaling=2^0
  GlissArr : Outport  Port=2  OutDataType=sfix(16)  OutScaling=2^0
  BetaObj : Outport  Port=3  OutDataType=sfix(16)  OutScaling=2^0
  ObsElat : Outport  Port=4  OutDataType=sfix(16)  OutScaling=2^0
  ObsElat1 : Outport  Port=5  OutDataType=sfix(16)  OutScaling=2^0
  wires:
  Discrete Derivative/1 -> Mux/2
  AngleBraquageArr/1 -> Mux/8
  Demux2/2 -> Mux/10
  Demux2/1 -> Mux/9
  Memory2/1 -> Demux2/1
  Gain2/1 -> ObsElat1/1
  Elat/1 -> Discrete Derivative/1, Mux/1
  Ecap/1 -> Discrete Derivative1/1, Mux/3, Mux2/2
  Mux/1 -> DetectGlissement/1
  DetectGlissement/1 -> Demux1/1
  Mux1/1 -> Memory2/1
  Demux1/1 -> GlissAv/1
  Demux1/2 -> GlissArr/1
  Courbure/1 -> Mux/5
  Vitesse/1 -> Mux/6
  AngleBraquage/1 -> Mux/7
  Demux1/4 -> Mux1/1, ObsElat/1
  Demux1/5 -> Mux1/2, Gain2/1, Mux2/1
  Demux1/3 -> BetaObj/1
  Discrete Derivative1/1 -> Mux/4
  Mux2/1 -> Scope/1

== system MotionControlRobuFastObsDynWithPredAdams2/ExtractionCourburePred/Point plus proche ==
  In1 : Inport  OutDataType=sfix(16)  OutScaling=2^0
  Memory : Memory  Orientation=left  X0=1  InheritSampleTime=on
  Mux2 : Mux  Inputs=2
  Point plus proche : MATLABFcn  MATLABFcn=point_plus_proche(u(1:2),u(3))  OutputDimensions=1  OutputSignalType=real  SampleTime=0.05
  Out1 : Outport  OutDataType=sfix(16)  OutScaling=2^0
  wires:
  Mux2/1 -> Point plus proche/1
  Point plus proche/1 -> Memory/1, Out1/1
  Memory/1 -> Mux2/2
  In1/1 -> Mux2/1

== system MotionControlRobuFastObsDynWithPredAdams2/ExtractionEtat/CorrPente ==
  In1 : Inport
  Demux : Demux  Outputs=2
  Divide1 : Product  Inputs=*/  OutDataType=sfix(16)  OutScaling=2^-10
  Divide2 : Product  Inputs=**  OutDataType=sfix(16)  OutScaling=2^-10
  Divide3 : Product  Inputs=**  OutDataType=sfix(16)  OutScaling=2^-10
  Divide4 : Product  Inputs=**  OutDataType=sfix(16)  OutScaling=2^-10
  Trigonometric Function1 : Trigonometry  Operator=cos
  Trigonometric Function2 : Trigonometry  Operator=cos
  Trigonometric Function3 : Trigonometry
  Trigonometric Function4 : Trigonometry  Operator=asin
  Trigonometric Function5 : Trigonometry  Operator=cos
  Out1 : Outport
  Out2 : Outport  Port=2
  wires:
  In1/1 -> Demux/1
  Demux/1 -> Divide1/1
  [Roulis] -> Trigonometric Function1/1
  Trigonometric Function1/1 -> Divide2/1, Divide3/2
  Trigonometric Function2/1 -> Divide2/2
  Divide2/1 -> Divide1/2
  Demux/2 -> Trigonometric Function2/1, Trigonometric Function3/1
  Divide4/1 -> Out1/1
  Divide1/1 -> Divide4/1
  Trigonometric Function3/1 -> Divide3/1
  Divide3/1 -> Trigonometric Function4/1
  Trigonometric Function4/1 -> Out2/1, Trigonometric Function5/1
  Trigonometric Function5/1 -> Divide4/2

== system MotionControlRobuFastObsDynWithPredAdams2/ExtractionEtat/Point plus proche ==
  In1 : Inport  OutDataType=sfix(16)  OutScaling=2^0
  Memory : Memory  Orientation=left  InheritSampleTime=on
  Mux2 : Mux  Inputs=2
  Point plus proche : MATLABFcn  MATLABFcn=point_plus_proche(u(1:3),u(4))  OutputDimensions=1  OutputSignalType=real  SampleTime=0.05
  Out1 : Outport  OutDataType=sfix(16)  OutScaling=2^0
  wires:
  Mux2/1 -> Point plus proche/1
  Point plus proche/1 -> Memory/1, Out1/1
  Memory/1 -> Mux2/2
  In1/1 -> Mux2/1

== system MotionControlRobuFastObsDynWithPredAdams2/ExtractionEtat/Retard2 ==
  In1 : Inport  OutDataType=sfix(16)  OutScaling=2^0
  Corr1 : Subsystem
  CorrPente : Subsystem
  Demux : Demux  Outputs=3
  Memory{1..4} (4 alike) : Memory  InheritSampleTime=on
  Mux1 : Mux  Inputs=3
  Out1 : Outport  OutDataType=sfix(16)  OutScaling=2^0
  wires:
  In1/1 -> Demux/1
  Demux/2 -> Mux1/2
  Demux/1 -> Mux1/1
  Mux1/1 -> Out1/1
  Demux/3 -> Corr1/1(In1)
  Corr1/1(Out1) -> Memory2/1
  Memory1/1 -> Memory4/1
  Memory2/1 -> Mux1/3

== system MotionControlRobuFastObsDynWithPredAdams2/Mesure/Bruit ==
  In1 : Inport  OutDataType=sfix(16)  OutScaling=2^0
  Random Number1 : RandomNumber  Variance=(0.1/3)^2  Seed=87  SampleTime=0.05
  Random Number2 : RandomNumber  Variance=0.0007  SampleTime=0.025
  Sum1 : Sum  OutDataType=sfix(16)  OutScaling=2^0
  Sum2 : Sum  OutDataType=sfix(16)  OutScaling=2^0
  Out1 : Outport  OutDataType=sfix(16)  OutScaling=2^0
  wires:
  Sum1/1 -> Out1/1
  In1/1 -> Sum1/1
  Random Number2/1 -> Sum1/2

== system MotionControlRobuFastObsDynWithPredAdams2/Mesure/Bruit1 ==
  In1 : Inport  OutDataType=sfix(16)  OutScaling=2^0
  Random Number1 : RandomNumber  Variance=(0.1/3)^2  Seed=75  SampleTime=0.05
  Random Number2 : RandomNumber  Variance=0.0007  SampleTime=0.025
  Sum1 : Sum  OutDataType=sfix(16)  OutScaling=2^0
  Sum2 : Sum  OutDataType=sfix(16)  OutScaling=2^0
  Out1 : Outport  OutDataType=sfix(16)  OutScaling=2^0
  wires:
  Random Number2/1 -> Sum1/2
  In1/1 -> Sum1/1
  Sum1/1 -> Out1/1

== system MotionControlRobuFastObsDynWithPredAdams2/Mesure/Bruit2 ==
  In1 : Inport  OutDataType=sfix(16)  OutScaling=2^0
  Random Number1 : RandomNumber  Variance=((1/3)*pi/180)^2  Seed=5  SampleTime=0.05
  Random Number2 : RandomNumber  Variance=0.0007  SampleTime=0.025
  Sum1 : Sum  OutDataType=sfix(16)  OutScaling=2^0
  Sum2 : Sum  OutDataType=sfix(16)  OutScaling=2^0
  Out1 : Outport  OutDataType=sfix(16)  OutScaling=2^0
  wires:
  Sum1/1 -> Out1/1
  In1/1 -> Sum1/1
  Random Number2/1 -> Sum1/2

== system MotionControlRobuFastObsDynWithPredAdams2/Mesure/Bruit3 ==
  In1 : Inport  OutDataType=sfix(16)  OutScaling=2^0
  Random Number1 : RandomNumber  Variance=((.1/3)*pi/180)^2  Seed=12  SampleTime=0.05
  Random Number2 : RandomNumber  Variance=0.0007  SampleTime=0.025
  Sum1 : Sum  OutDataType=sfix(16)  OutScaling=2^0
  Sum2 : Sum  OutDataType=sfix(16)  OutScaling=2^0
  Out1 : Outport  OutDataType=sfix(16)  OutScaling=2^0
  wires:
  Random Number2/1 -> Sum1/2
  In1/1 -> Sum1/1
  Sum1/1 -> Out1/1

== system MotionControlRobuFastObsDynWithPredAdams2/Mesure/Bruit4 ==
  In1 : Inport  OutDataType=sfix(16)  OutScaling=2^0
  Random Number1 : RandomNumber  Variance=((.1/3)*pi/180)^2  Seed=12  SampleTime=0.05
  Random Number2 : RandomNumber  Variance=0.0007  SampleTime=0.025
  Sum1 : Sum  OutDataType=sfix(16)  OutScaling=2^0
  Sum2 : Sum  OutDataType=sfix(16)  OutScaling=2^0
  Out1 : Outport  OutDataType=sfix(16)  OutScaling=2^0
  wires:
  Sum1/1 -> Out1/1
  In1/1 -> Sum1/1
  Random Number2/1 -> Sum1/2

== system MotionControlRobuFastObsDynWithPredAdams2/Mesure/Retard1 ==
  In1 : Inport  OutDataType=sfix(16)  OutScaling=2^0
  Memory1 : Memory  InheritSampleTime=on
  Memory4 : Memory  InheritSampleTime=on
  Out1 : Outport  OutDataType=sfix(16)  OutScaling=2^0
  wires:
  In1/1 -> Memory4/1
  Memory4/1 -> Memory1/1
  Memory1/1 -> Out1/1

== system MotionControlRobuFastObsDynWithPredAdams2/RobuFAST1/Bruit2 ==
  In1 : Inport  OutDataType=sfix(16)  OutScaling=2^0
  Random Number1 : RandomNumber  Mean=4*pi/180  Variance=((5/3)*pi/180)^2  Seed=15  SampleTime=0.05
  Random Number2 : RandomNumber  Variance=0.0007  SampleTime=0.025
  Sum1 : Sum  OutDataType=sfix(16)  OutScaling=2^0
  Sum2 : Sum  OutDataType=sfix(16)  OutScaling=2^0
  Out1 : Outport  OutDataType=sfix(16)  OutScaling=2^0
  wires:
  Sum1/1 -> Out1/1
  In1/1 -> Sum1/1
  Random Number2/1 -> Sum1/2

== system MotionControlRobuFastObsDynWithPredAdams2/RobuFAST1/Corr1 ==
  In1 : Inport
  MATLAB Fcn : MATLABFcn  MATLABFcn=Corr180(u(1))  OutputDimensions=1  SampleTime=0.05
  Out1 : Outport
  wires:
  In1/1 -> MATLAB Fcn/1
  MATLAB Fcn/1 -> Out1/1

== system MotionControlRobuFastObsDynWithPredAdams2/RobuFAST1/CorrPente ==
  In1 : Inport
  Divide3 : Product  Inputs=**  OutDataType=sfix(16)  OutScaling=2^-10
  Trigonometric Function2 : Trigonometry  Operator=cos
  Out1 : Outport
  wires:
  In1/1 -> Divide3/1
  [Roulis] -> Trigonometric Function2/1
  Trigonometric Function2/1 -> Divide3/2
  Divide3/1 -> Out1/1

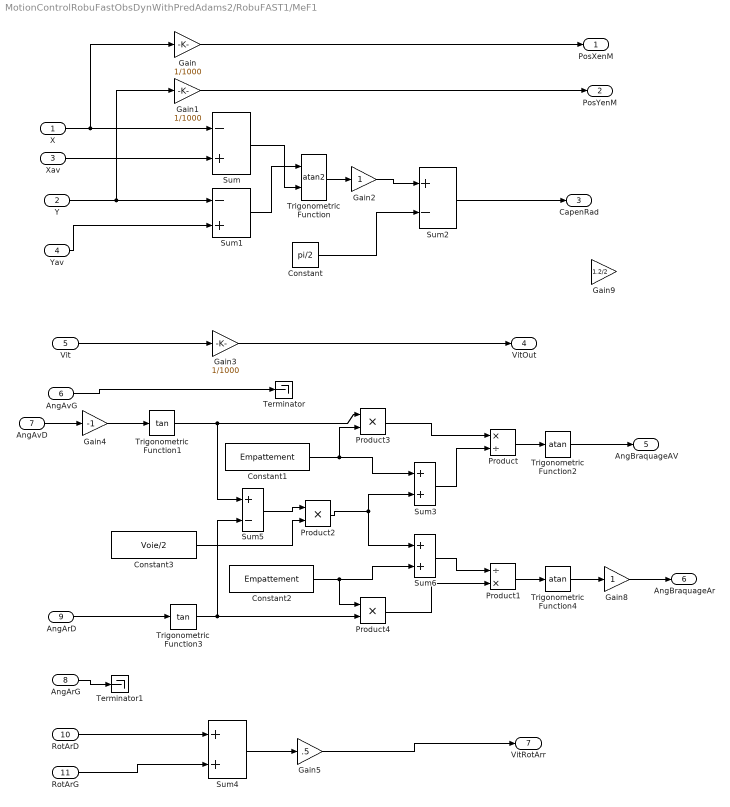
== system MotionControlRobuFastObsDynWithPredAdams2/RobuFAST1/MeF1 ==
  X : Inport  OutDataType=sfix(16)  OutScaling=2^0
  Y : Inport  Port=2  OutDataType=sfix(16)  OutScaling=2^0
  Xav : Inport  Port=3  OutDataType=sfix(16)  OutScaling=2^0
  Yav : Inport  Port=4  OutDataType=sfix(16)  OutScaling=2^0
  Vit : Inport  Port=5  OutDataType=sfix(16)  OutScaling=2^0
  AngAvG : Inport  Port=6  OutDataType=sfix(16)  OutScaling=2^0
  AngAvD : Inport  Port=7  OutDataType=sfix(16)  OutScaling=2^0
  AngArG : Inport  Port=8  OutDataType=sfix(16)  OutScaling=2^0
  AngArD : Inport  Port=9  OutDataType=sfix(16)  OutScaling=2^0
  RotArD : Inport  Port=10  OutDataType=sfix(16)  OutScaling=2^0
  RotArG : Inport  Port=11  OutDataType=sfix(16)  OutScaling=2^0
  Constant : Constant  Value=pi/2  OutDataType=sfix(16)  OutScaling=2^0
  Constant1 : Constant  Value=Empattement  OutDataType=sfix(16)  OutScaling=2^0
  Constant2 : Constant  Value=Empattement  OutDataType=sfix(16)  OutScaling=2^0
  Constant3 : Constant  Value=Voie/2  OutDataType=sfix(16)  OutScaling=2^0
  Gain : Gain  Gain=1/1000  ParameterDataType=sfix(16)  ParameterScaling=2^0  OutDataType=sfix(16)  OutScaling=2^0
  Gain1 : Gain  Gain=1/1000  ParameterDataType=sfix(16)  ParameterScaling=2^0  OutDataType=sfix(16)  OutScaling=2^0
  Gain2 : Gain  ParameterDataType=sfix(16)  ParameterScaling=2^0  OutDataType=sfix(16)  OutScaling=2^0
  Gain3 : Gain  Gain=1/1000  ParameterDataType=sfix(16)  ParameterScaling=2^0  OutDataType=sfix(16)  OutScaling=2^0
  Gain4 : Gain  Gain=-1  ParameterDataType=sfix(16)  ParameterScaling=2^0  OutDataType=sfix(16)  OutScaling=2^0
  Gain5 : Gain  Gain=.5  ParameterDataType=sfix(16)  ParameterScaling=2^0  OutDataType=sfix(16)  OutScaling=2^0
  Gain8 : Gain  ParameterDataType=sfix(16)  ParameterScaling=2^0  OutDataType=sfix(16)  OutScaling=2^0
  Gain9 : Gain  Gain=1.2/2  ParameterDataType=sfix(16)  ParameterScaling=2^0  OutDataType=sfix(16)  OutScaling=2^0
  Product : Product  Inputs=*/  OutDataType=sfix(16)  OutScaling=2^0  RndMeth=Zero
  Product1 : Product  Inputs=/*  OutDataType=sfix(16)  OutScaling=2^0  RndMeth=Zero
  Product2 : Product  Inputs=**  OutDataType=sfix(16)  OutScaling=2^0  RndMeth=Zero
  Product3 : Product  Inputs=**  OutDataType=sfix(16)  OutScaling=2^0  RndMeth=Zero
  Product4 : Product  Inputs=**  OutDataType=sfix(16)  OutScaling=2^0  RndMeth=Zero
  Sum : Sum  Inputs=-+  OutDataType=sfix(16)  OutScaling=2^0
  Sum1 : Sum  Inputs=-+  OutDataType=sfix(16)  OutScaling=2^0
  Sum2 : Sum  Inputs=+-  OutDataType=sfix(16)  OutScaling=2^0
  Sum3 : Sum  OutDataType=sfix(16)  OutScaling=2^0
  Sum4 : Sum  OutDataType=sfix(16)  OutScaling=2^0
  Sum5 : Sum  Inputs=+-  OutDataType=sfix(16)  OutScaling=2^0
  Sum6 : Sum  OutDataType=sfix(16)  OutScaling=2^0
  Terminator : Terminator
  Terminator1 : Terminator
  Trigonometric Function : Trigonometry  Operator=atan2
  Trigonometric Function1 : Trigonometry  Operator=tan
  Trigonometric Function2 : Trigonometry  Operator=atan
  Trigonometric Function3 : Trigonometry  Operator=tan
  Trigonometric Function4 : Trigonometry  Operator=atan
  PosXenM : Outport  OutDataType=sfix(16)  OutScaling=2^0
  PosYenM : Outport  Port=2  OutDataType=sfix(16)  OutScaling=2^0
  CapenRad : Outport  Port=3  OutDataType=sfix(16)  OutScaling=2^0
  VitOut : Outport  Port=4  OutDataType=sfix(16)  OutScaling=2^0
  AngBraquageAV : Outport  Port=5  OutDataType=sfix(16)  OutScaling=2^0
  AngBraquageAr : Outport  Port=6  OutDataType=sfix(16)  OutScaling=2^0
  VitRotArr : Outport  Port=7  OutDataType=sfix(16)  OutScaling=2^0
  wires:
  X/1 -> Sum/1, Gain/1
  Y/1 -> Sum1/1, Gain1/1
  Xav/1 -> Sum/2
  Trigonometric Function/1 -> Gain2/1
  Yav/1 -> Sum1/2
  Gain1/1 -> PosYenM/1
  Gain2/1 -> Sum2/1
  Constant/1 -> Sum2/2
  Sum2/1 -> CapenRad/1
  Vit/1 -> Gain3/1
  Gain3/1 -> VitOut/1
  AngAvD/1 -> Gain4/1
  Sum4/1 -> Gain5/1
  RotArD/1 -> Sum4/1
  RotArG/1 -> Sum4/2
  Gain5/1 -> VitRotArr/1
  AngArD/1 -> Trigonometric Function3/1
  AngAvG/1 -> Terminator/1
  Trigonometric Function1/1 -> Sum5/1, Product3/1
  Sum3/1 -> Product/2
  Product3/1 -> Product/1
  Product/1 -> Trigonometric Function2/1
  Trigonometric Function2/1 -> AngBraquageAV/1
  AngArG/1 -> Terminator1/1
  Trigonometric Function3/1 -> Sum5/2, Product4/2
  Constant1/1 -> Sum3/1, Product3/2
  Sum5/1 -> Product2/1
  Product2/1 -> Sum3/2, Sum6/1
  Sum6/1 -> Product1/1
  Product4/1 -> Product1/2
  Constant2/1 -> Sum6/2, Product4/1
  Product1/1 -> Trigonometric Function4/1
  Trigonometric Function4/1 -> Gain8/1
  Gain8/1 -> AngBraquageAr/1
  Sum1/1 -> Trigonometric Function/1
  Sum/1 -> Trigonometric Function/2
  Gain/1 -> PosXenM/1
  Constant3/1 -> Product2/2
  Gain4/1 -> Trigonometric Function1/1

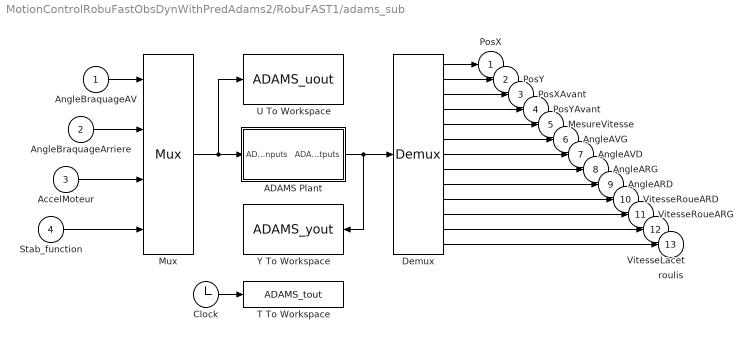
== system MotionControlRobuFastObsDynWithPredAdams2/RobuFAST1/adams_sub ==
  "AngleBraquageAV     " : Inport
  AngleBraquageArriere : Inport  Port=2
  "AccelMoteur         " : Inport  Port=3
  "Stab_function       " : Inport  Port=4
  ADAMS Plant : Subsystem  mask(Adams Plant){exevie=ADAMS_sysdir, workdir=ADAMS_cwd, comtyp=PIPE(DDE), ada_host=ADAMS_host, exetyp=C++, exesol=ADAMS_exec, nampre=ADAMS_prefix, nam_in=ADAMS_inputs, namout=ADAMS_outputs, outfil=ADAMS_prefix, dt_out=0.01, o_rate=1, interorder=0, dft=no, modsim=discrete, modani=interactive, stat=ADAMS_static, inicmd=[ADAMS_init]}
      mask prompts: exevie "Adams install directory"; workdir "Adams working directory"; comtyp "Interprocess Option"; ada_host "Adams host"; exetyp "Adams solver type"; exesol "User executable (opt.: if blank - use standard)"; nampre "Adams model file prefix"; nam_in "Adams/View input names"; namout "Adams/View output names"; outfil "Output files prefix (opt.: if blank - no output)"; dt_out "Communication Interval"; o_rate "Number of communications per output step"; interorder "Interpolation Order"; dft "Direct Feedthrough"; modsim "Simulation     mode"; modani "Animation     mode"; stat "Initial Static Simulation Flag"; inicmd "Initialization commands"
      mask help: Simulate any Adams plant model either in Adams/Solver form (.adm file) or in Adams/View form (.cmd file)
      mask StyleString: edit,edit,popup(PIPE(DDE)|TCP/IP),edit,popup(Fortran|C++),edit,edit,edit,edit,edit,edit,edit,edit,popup(no|yes),popup(discrete|continuous),popup(batch|interactive),edit,edit
      mask Display: disp( 'MSCSoftware' )
  Clock : Clock
      settings: Decimation=10
  Demux : Demux  Outputs=13
  Mux : Mux
  T To Workspace : ToWorkspace  VariableName=ADAMS_tout  SaveFormat=Array
      settings: MaxDataPoints=100000
  U To Workspace : ToWorkspace  VariableName=ADAMS_uout  SaveFormat=Array
      settings: MaxDataPoints=100000
  Y To Workspace : ToWorkspace  VariableName=ADAMS_yout  SaveFormat=Array
      settings: MaxDataPoints=100000
  "PosX          " : Outport
  "PosY          " : Outport  Port=2
  "PosXAvant     " : Outport  Port=3
  "PosYAvant     " : Outport  Port=4
  "MesureVitesse " : Outport  Port=5
  "AngleAVG      " : Outport  Port=6
  "AngleAVD      " : Outport  Port=7
  "AngleARG      " : Outport  Port=8
  "AngleARD      " : Outport  Port=9
  VitesseRoueARD : Outport  Port=10
  VitesseRoueARG : Outport  Port=11
  "VitesseLacet  " : Outport  Port=12
  "roulis        " : Outport  Port=13
  wires:
  Clock/1 -> T To Workspace/1
  Mux/1 -> ADAMS Plant/1(ADAMS inputs), U To Workspace/1
  ADAMS Plant/1(ADAMS outputs) -> Demux/1, Y To Workspace/1
  Demux/1 -> "PosX          "/1
  Demux/2 -> "PosY          "/1
  Demux/3 -> "PosXAvant     "/1
  Demux/4 -> "PosYAvant     "/1
  Demux/5 -> "MesureVitesse "/1
  Demux/6 -> "AngleAVG      "/1
  Demux/7 -> "AngleAVD      "/1
  Demux/8 -> "AngleARG      "/1
  Demux/9 -> "AngleARD      "/1
  Demux/10 -> VitesseRoueARD/1
  Demux/11 -> VitesseRoueARG/1
  Demux/12 -> "VitesseLacet  "/1
  Demux/13 -> "roulis        "/1
  "AngleBraquageAV     "/1 -> Mux/1
  AngleBraquageArriere/1 -> Mux/2
  "AccelMoteur         "/1 -> Mux/3
  "Stab_function       "/1 -> Mux/4

== system MotionControlRobuFastObsDynWithPredAdams2/CommandeAvGlissement1/ExtractionRigid/Subsystem ==
  In1 : Inport
  Memory{1..5,7..11} (10 alike) : Memory  InheritSampleTime=on
  Out1 : Outport
  wires:
  Memory7/1 -> Memory8/1
  Memory8/1 -> Memory9/1
  Memory9/1 -> Memory10/1
  Memory10/1 -> Memory11/1
  In1/1 -> Memory7/1
  Memory3/1 -> Memory4/1
  Memory4/1 -> Memory5/1
  Memory5/1 -> Memory1/1
  Memory1/1 -> Memory2/1
  Memory11/1 -> Memory3/1
  Memory2/1 -> Out1/1

== system MotionControlRobuFastObsDynWithPredAdams2/CommandeAvGlissement1/ExtractionRigid/Subsystem2 ==
  In1 : Inport
  Memory{1..5,7..11} (10 alike) : Memory  InheritSampleTime=on
  Out1 : Outport
  wires:
  Memory2/1 -> Out1/1
  Memory11/1 -> Memory3/1
  Memory1/1 -> Memory2/1
  Memory5/1 -> Memory1/1
  Memory4/1 -> Memory5/1
  Memory3/1 -> Memory4/1
  In1/1 -> Memory7/1
  Memory10/1 -> Memory11/1
  Memory9/1 -> Memory10/1
  Memory8/1 -> Memory9/1
  Memory7/1 -> Memory8/1
